simulink model "rlWalkingBipedRobot"  (R2023b)
settings: Solver=ode23t  StartTime=0.0  StopTime=inf  RelTol=1e-2  EnableMultiTasking=on
undefined symbols (not defined in the file): height_plane, init_angs_L, init_angs_R, init_height, joint_stiffness, lower_leg_length, max_torque, plane_x, plane_y, Tf, torso_offset_x, torso_offset_z, torso_x, torso_y, torso_z, Ts, upper_leg_length, wx0, wy0, X, Y, Z
libraries: sm_lib x27, nesl_utility x14, walkingRobotUtils x10, simulink x5, rllib x1
(part 2 of 2)

== system rlWalkingBipedRobot/Walking Robot/World and Ground ==
  Mechanism Configuration : sm_lib/Utilities/Mechanism Configuration  UniformGravity=Constant  GravityVector=[0 0 -9.80665]  GravityVectorUnits=m/s^2  LinearizationDelta=0.001  JointModeTransitionNonlinearIterations=2
  Plane Offset : sm_lib/Frames and Transforms/Rigid Transform  TranslationMethod=StandardAxis  TranslationStandardOffset=height_plane/2  TranslationStandardOffsetUnits=m  TranslationStandardAxis=-Z  TranslationCartesianOffset=[0 0 0]  TranslationCartesianOffsetUnits=m  TranslationROffset=0  TranslationROffsetUnits=m  TranslationZOffset=0  TranslationZOffsetUnits=m  TranslationThetaOffset=0  TranslationThetaOffsetUnits=deg  RotationMethod=None  RotationAngleUnits=deg  RotationStandardAxis=+Z  RotationAngle=0.0  RotationArbitraryAxis=[0 0 1]  FollAlignAxisA=+X  BaseAlignAxisA=+Y  FollAlignAxisB=+Y  BaseAlignAxisB=+Z  RotationSequenceAxes=FollowerAxes  RotationSequence=XYX  RotationSequenceAngles=[0 0 0]  RotationSequenceAnglesUnits=deg  RotationMatrix=[1 0 0; 0 1 0; 0 0 1]  Quaternion=[1 0 0 0]
  Solver Configuration : nesl_utility/Solver Configuration  PhysicalDomain=network_engine_domain  SubClassName=solver  LeftPortType=input  RightPortType=generic  Tones=[]  Harmonics=[]  SimulateNoise=off  Profile=off  UseLocalSampling=off  EnableSwitchedLinearOptims=on  FrequencyDomain=off  UseCCode=off  RelTol=0.001  AbsTol=1e-06  MinStep=1e-09  ToWorkspace=off  RevertToSquareIcSolve=off  NumHomotopyIterations=100  PhasorMode=off  PhasorModeNumHarmonics=1  ConsistencySolver=NEWTON_FTOL  IndexReductionMethod=DerivativeReplacement  DoDC=off  ResidualTolerance=1e-09  ConsistencyTolSource=GLOBAL  ConsistencyAbsTol=0.001  ConsistencyRelTol=0.001  ConsistencyTolFactor=0.001  UseLocalSolver=off  LocalSolverChoice=NE_TRAPEZOIDAL_ADVANCER  ResolveIndetEquations=on  FunctionEvalNumThread=1  LocalSolverSampleTime=Ts  DoFixedCost=off  MaxNonlinIter=3  MaxModeIter=2  ComputeImpulses=off  ImpulseIterations=2  LinearAlgebra=Sparse  LinearAlgebraNumThread=0  EquationFormulation=NE_TIME_EF  DelaysMemoryBudget=1024  AutomaticFiltering=on  FilteringTimeConstant=0.001  PartitionStorageMethod=AS_NEEDED  PartitionMemoryBudget=1024  PartitionMethod=FAST  MultibodyUseLocalSolver=off  MultibodyLocalSolverChoice=ODE1  MultibodyLocalSolverSampleTime=0.001
  World Frame1 : sm_lib/Frames and Transforms/World Frame
  World Plane : sm_lib/Body Elements/Brick Solid  GraphicAmbientColor=[0.15 0.15 0.15 1.0]  BasedOnType=Density  BrickDimensions="[plane_x plane_y  height_plane]"  BrickDimensionsUnits=m  CenterOfMass=[0 0 0]  CenterOfMassUnits=m  GraphicDiffuseColor=[1.0 1.0 0.8]  Density=density  DensityUnits=kg/(m^3)  DoExposeReferenceFrame=on  GraphicEmissiveColor=[0.0 0.0 0.0 1.0]  ExportEntireGeometry=on  SerializedFrames=<Frames/>  MarkerShape=Sphere  MarkerSize=10  GraphicType=FromGeometry  InertiaType=CalculateFromGeometry  Mass=1  MassUnits=kg  MomentsOfInertia=[1 1 1]  MomentsOfInertiaUnits=kg*m^2  GraphicOpacity=0.5  ProductsOfInertia=[0 0 0]  ProductsOfInertiaUnits=kg*m^2  GraphicShininess=75  GraphicSpecularColor=[0.5 0.5 0.5 1.0]  GraphicVisPropType=SimpleVisualProperties
  W : PMIOPort  Side=Left
  G : PMIOPort  Port=2  Side=Right
  connections:
  G/RConn1 -- World Plane/LConn1
  World Plane/RConn1 -- Plane Offset/RConn1
  Solver Configuration/RConn1 -- Plane Offset/LConn1 -- Mechanism Configuration/RConn1 -- W/RConn1 -- World Frame1/RConn1

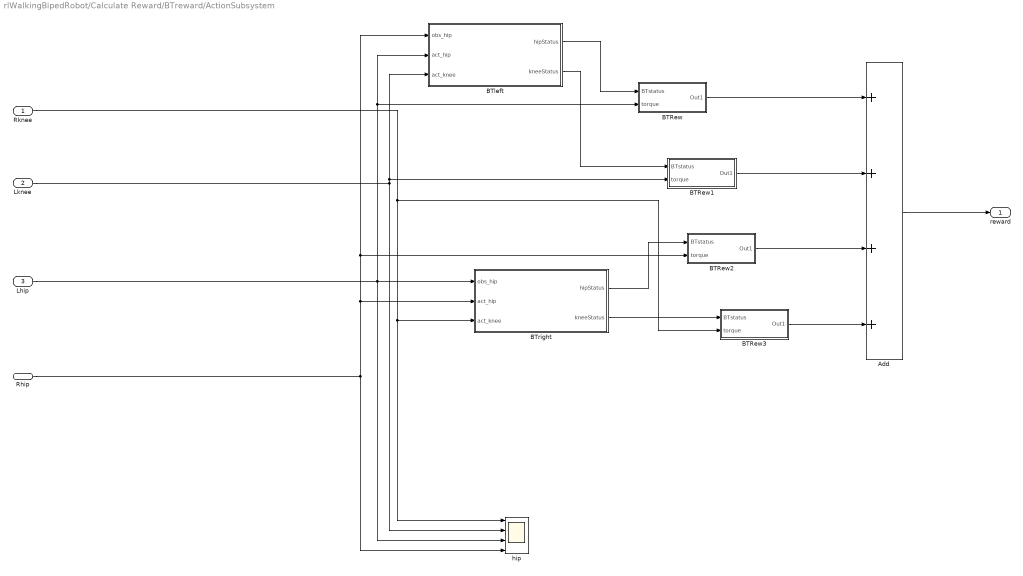
== system rlWalkingBipedRobot/Calculate Reward/BTreward/ActionSubsystem ==
  Rknee : Inport
  Lknee : Inport  Port=2
  Lhip : Inport  Port=3
  Rhip : Inport  Port=4
  Add : Sum  Inputs=++++
  BTRew : Subsystem
  BTRew1 : Subsystem
  BTRew2 : Subsystem
  BTRew3 : Subsystem
  BTleft : Subsystem
  BTright : Subsystem
  hip : Scope  NumInputPorts=4
  reward : Outport
  wires:
  Rknee/1 -> BTright/3(act_knee), hip/1, BTRew3/2(torque)
  Lknee/1 -> BTRew1/2(torque), BTleft/3(act_knee), hip/2
  Lhip/1 -> BTleft/2(act_hip), BTRew/2(torque), BTright/1(obs_hip), hip/3
  Rhip/1 -> BTRew2/2(torque), BTleft/1(obs_hip), BTright/2(act_hip), hip/4
  BTleft/1(hipStatus) -> BTRew/1(BTstatus)
  BTleft/2(kneeStatus) -> BTRew1/1(BTstatus)
  BTright/1(hipStatus) -> BTRew2/1(BTstatus)
  BTright/2(kneeStatus) -> BTRew3/1(BTstatus)
  BTRew/1(Out1) -> Add/1
  BTRew1/1(Out1) -> Add/2
  BTRew2/1(Out1) -> Add/3
  BTRew3/1(Out1) -> Add/4
  Add/1 -> reward/1

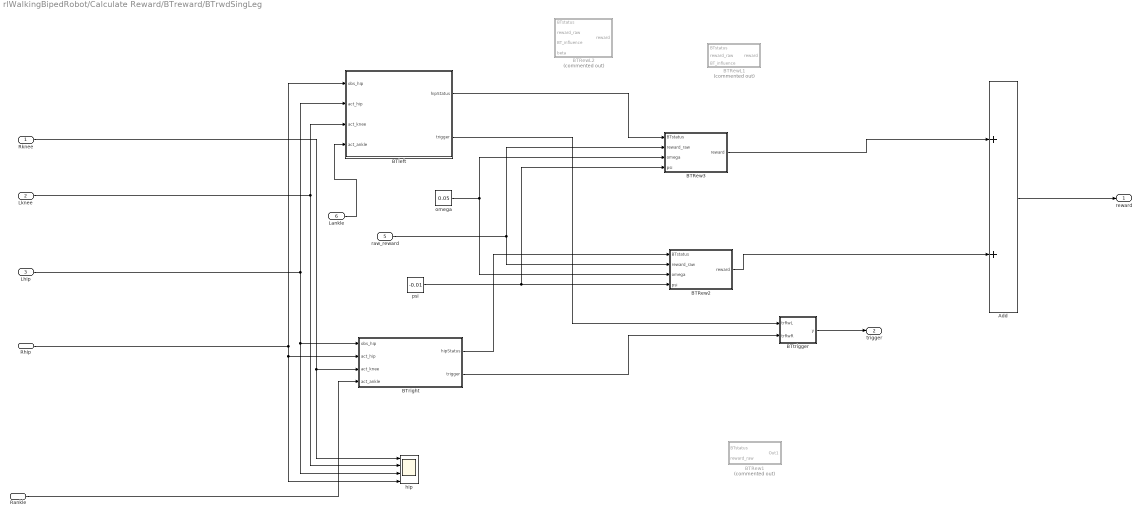
== system rlWalkingBipedRobot/Calculate Reward/BTreward/BTrwdSingLeg ==
  Rknee : Inport
  Lknee : Inport  Port=2
  Lhip : Inport  Port=3
  Rhip : Inport  Port=4
  raw_reward : Inport  Port=5
  Lankle : Inport  Port=6
  Rankle : Inport  Port=7
  Add : Sum
  BTRew1 : Subsystem  Commented=on
  BTRew2 : Subsystem
  BTRew3 : Subsystem
  BTRewL1 : Subsystem  Commented=on
  BTRewL2 : Subsystem  Commented=on
  BTleft : Subsystem
  BTright : Subsystem
  BTtrigger : MATLAB Function  TreatAsAtomicUnit=on
  hip : Scope  NumInputPorts=4
  omega : Constant  Value=0.05
  psi : Constant  Value=-0.01
  reward : Outport
  trigger : Outport  Port=2
  wires:
  Rknee/1 -> hip/1, BTright/3(act_knee)
  Lknee/1 -> BTleft/3(act_knee), hip/2
  Lhip/1 -> hip/3, BTright/1(obs_hip), BTleft/2(act_hip)
  Rhip/1 -> hip/4, BTright/2(act_hip), BTleft/1(obs_hip)
  BTRew3/1(reward) -> Add/1
  BTRew2/1(reward) -> Add/2
  Add/1 -> reward/1
  raw_reward/1 -> BTRew3/2(reward_raw), BTRew2/2(reward_raw)
  BTtrigger/1(y) -> trigger/1
  BTleft/1(hipStatus) -> BTRew3/1(BTstatus)
  BTright/1(hipStatus) -> BTRew2/1(BTstatus)
  BTleft/2(trigger) -> BTtrigger/1(trRwL)
  BTright/2(trigger) -> BTtrigger/2(trRwR)
  Rankle/1 -> BTright/4(act_ankle)
  Lankle/1 -> BTleft/4(act_ankle)
  omega/1 -> BTRew3/3(omega), BTRew2/3(omega)
  psi/1 -> BTRew3/4(psi), BTRew2/4(psi)

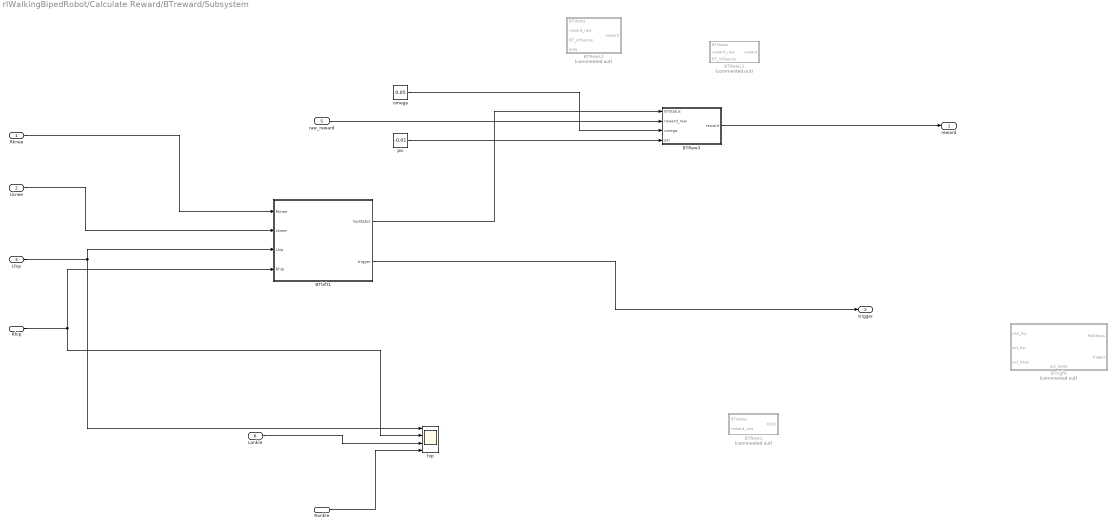
== system rlWalkingBipedRobot/Calculate Reward/BTreward/Subsystem ==
  Rknee : Inport
  Lknee : Inport  Port=2
  Lhip : Inport  Port=3
  Rhip : Inport  Port=4
  raw_reward : Inport  Port=5
  Lankle : Inport  Port=6
  Rankle : Inport  Port=7
  BTRew1 : Subsystem  Commented=on
  BTRew3 : Subsystem
  BTRewL1 : Subsystem  Commented=on
  BTRewL2 : Subsystem  Commented=on
  BTleft1 : Subsystem
  BTright : Subsystem  Commented=on
      settings: PortSchema="{\"entries\":[{\"content\":{\"sides\":[{\"content\":{\"connectorIds\":[\"In1\",\"In2\",\"In3\"]},\"type\":\"ConnectorPlacement.EquallySpacedRectSide\",\"uuid\":\"d1a7c831-0d82-4d6a-8038-37bdddb40f4b\"},{\"content\":{\"connectorIds\":[\"Out1\",\"Out2\"],\"side\":\"RIGHT\"},\"type\":\"ConnectorPlacement.EquallySpacedRectSide\",\"uuid\":\"e646f7d3-ea41-40b5-b80d-dc533f9acebb\"},{\"content\":{\"side\":\"TOP\"},\"type\":\"ConnectorPlacement.EquallySpacedRectSide\",\"uuid\":\"96bfc05b-3d35-40ea-a71c-eb204fc643e2\"},{\"content\":{\"connectorIds\":[\"In4\"],\"side\":\"BOTTOM\"},\"type\":\"ConnectorPlacement.EquallySpacedRectSide\",\"uuid\":\"1094da1b-3afd-404e-9933-6191ea7e4b5f\"}]},\"type\":\"ConnectorPlacement.EquallySpacedConnector\",\"uuid\":\"abf6e411-f407-44d6-9c89-b64076b2e2db\"}],\"packageUris\":[\"http://schema.mathworks.com/mf0/Connector/R2020b\"],\"version\":\"1.0\"}"
  hip : Scope  NumInputPorts=4
  omega : Constant  Value=0.05
  psi : Constant  Value=-0.01
  reward : Outport
  trigger : Outport  Port=2
  wires:
  Rknee/1 -> BTleft1/1(Rknee)
  Lknee/1 -> BTleft1/2(Lknee)
  Lhip/1 -> hip/1, BTleft1/3(Lhip)
  Rhip/1 -> hip/2, BTleft1/4(Rhip)
  BTRew3/1(reward) -> reward/1
  raw_reward/1 -> BTRew3/2(reward_raw)
  BTleft1/2(trigger) -> trigger/1
  Lankle/1 -> hip/3
  omega/1 -> BTRew3/3(omega)
  psi/1 -> BTRew3/4(psi)
  BTleft1/1(hipStatus) -> BTRew3/1(BTstatus)
  Rankle/1 -> hip/4

== system rlWalkingBipedRobot/Walking Robot/Sensors/Calculate Actuator Power ==
  meas : Inport
  Add : Sum  Inputs=3
  Bus Selector : BusSelector  OutputSignals=ankle_speed,ankle_torque,knee_speed,knee_torque,hip_speed,hip_torque
  Product : Product
  Product1 : Product
  Product2 : Product
  P : Outport  VectorParamsAs1DForOutWhenUnconnected=off
  wires:
  meas/1 -> Bus Selector/1
  Product2/1 -> Add/3
  Product1/1 -> Add/2
  Product/1 -> Add/1
  Add/1 -> P/1
  Bus Selector/1 -> Product/1  "<ankle_speed>"
  Bus Selector/2 -> Product/2  "<ankle_torque>"
  Bus Selector/3 -> Product1/1  "<knee_speed>"
  Bus Selector/4 -> Product1/2  "<knee_torque>"
  Bus Selector/5 -> Product2/1  "<hip_speed>"
  Bus Selector/6 -> Product2/2  "<hip_torque>"

== system rlWalkingBipedRobot/Walking Robot/Sensors/Calculate Actuator Power1 ==
  meas : Inport
  Add : Sum  Inputs=3
  Bus Selector : BusSelector  OutputSignals=ankle_speed,ankle_torque,knee_speed,knee_torque,hip_speed,hip_torque
  Product : Product
  Product1 : Product
  Product2 : Product
  P : Outport  VectorParamsAs1DForOutWhenUnconnected=off
  wires:
  Bus Selector/6 -> Product2/2  "<hip_torque>"
  Bus Selector/5 -> Product2/1  "<hip_speed>"
  Bus Selector/4 -> Product1/2  "<knee_torque>"
  Bus Selector/3 -> Product1/1  "<knee_speed>"
  Bus Selector/2 -> Product/2  "<ankle_torque>"
  Bus Selector/1 -> Product/1  "<ankle_speed>"
  Add/1 -> P/1
  Product/1 -> Add/1
  Product1/1 -> Add/2
  Product2/1 -> Add/3
  meas/1 -> Bus Selector/1

== system rlWalkingBipedRobot/Calculate Reward/BTreward/ActionSubsystem/BTRew ==
  BTstatus : Inport
  torque : Inport  Port=2
  Abs : Abs  SaturateOnIntegerOverflow=off
  Gain : Gain  Gain=0.1
  Product : Product
  Out1 : Outport
  wires:
  Gain/1 -> Out1/1
  torque/1 -> Abs/1
  Abs/1 -> Product/2
  Product/1 -> Gain/1
  BTstatus/1 -> Product/1

== system rlWalkingBipedRobot/Calculate Reward/BTreward/ActionSubsystem/BTRew1 ==
  BTstatus : Inport
  torque : Inport  Port=2
  Abs : Abs  SaturateOnIntegerOverflow=off
  Gain : Gain  Gain=0.1
  Product : Product
  Out1 : Outport
  wires:
  Gain/1 -> Out1/1
  torque/1 -> Abs/1
  Abs/1 -> Product/2
  Product/1 -> Gain/1
  BTstatus/1 -> Product/1

== system rlWalkingBipedRobot/Calculate Reward/BTreward/ActionSubsystem/BTRew2 ==
  BTstatus : Inport
  torque : Inport  Port=2
  Abs : Abs  SaturateOnIntegerOverflow=off
  Gain : Gain  Gain=0.1
  Product : Product
  Out1 : Outport
  wires:
  Gain/1 -> Out1/1
  torque/1 -> Abs/1
  Abs/1 -> Product/2
  Product/1 -> Gain/1
  BTstatus/1 -> Product/1

== system rlWalkingBipedRobot/Calculate Reward/BTreward/ActionSubsystem/BTRew3 ==
  BTstatus : Inport
  torque : Inport  Port=2
  Abs : Abs  SaturateOnIntegerOverflow=off
  Gain : Gain  Gain=0.1
  Product : Product
  Out1 : Outport
  wires:
  Gain/1 -> Out1/1
  torque/1 -> Abs/1
  Abs/1 -> Product/2
  Product/1 -> Gain/1
  BTstatus/1 -> Product/1

== system rlWalkingBipedRobot/Calculate Reward/BTreward/ActionSubsystem/BTleft ==
  obs_hip : Inport
  act_hip : Inport  Port=2
  act_knee : Inport  Port=3
  BT : MATLAB Function  TreatAsAtomicUnit=on
  hipStatus : Outport
  kneeStatus : Outport  Port=2
  wires:
  obs_hip/1 -> BT/1(u)
  BT/1(y) -> hipStatus/1
  act_hip/1 -> BT/2(t)
  act_knee/1 -> BT/3(s)
  BT/2(z) -> kneeStatus/1

== system rlWalkingBipedRobot/Calculate Reward/BTreward/ActionSubsystem/BTright ==
  obs_hip : Inport
  act_hip : Inport  Port=2
  act_knee : Inport  Port=3
  BT : MATLAB Function  TreatAsAtomicUnit=on
  hipStatus : Outport
  kneeStatus : Outport  Port=2
  wires:
  obs_hip/1 -> BT/1(u)
  BT/1(y) -> hipStatus/1
  act_hip/1 -> BT/2(t)
  act_knee/1 -> BT/3(s)
  BT/2(z) -> kneeStatus/1

== system rlWalkingBipedRobot/Calculate Reward/BTreward/BTrwdSingLeg/BTRew1 ==
  BTstatus : Inport
  reward_raw : Inport  Port=2
  Product1 : Product
  rew2BT : MATLAB Function  TreatAsAtomicUnit=on
  Out1 : Outport
  wires:
  Product1/1 -> Out1/1
  BTstatus/1 -> Product1/1
  reward_raw/1 -> rew2BT/1(x)
  rew2BT/1(y) -> Product1/2

== system rlWalkingBipedRobot/Calculate Reward/BTreward/BTrwdSingLeg/BTRew2 ==
  BTstatus : Inport
  reward_raw : Inport  Port=2
  omega : Inport  Port=3
  psi : Inport  Port=4
  rew2BT : MATLAB Function  TreatAsAtomicUnit=on
  reward : Outport
  wires:
  rew2BT/1(y) -> reward/1
  BTstatus/1 -> rew2BT/3(BTstatus)
  reward_raw/1 -> rew2BT/4(x)
  omega/1 -> rew2BT/1(omega)
  psi/1 -> rew2BT/2(psi)

== system rlWalkingBipedRobot/Calculate Reward/BTreward/BTrwdSingLeg/BTRew3 ==
  BTstatus : Inport
  reward_raw : Inport  Port=2
  omega : Inport  Port=3
  psi : Inport  Port=4
  rew2BT : MATLAB Function  TreatAsAtomicUnit=on
  reward : Outport
  wires:
  rew2BT/1(y) -> reward/1
  BTstatus/1 -> rew2BT/3(BTstatus)
  reward_raw/1 -> rew2BT/4(x)
  omega/1 -> rew2BT/1(omega)
  psi/1 -> rew2BT/2(psi)

== system rlWalkingBipedRobot/Calculate Reward/BTreward/BTrwdSingLeg/BTRewL1 ==
  BTstatus : Inport
  reward_raw : Inport  Port=2
  BT_influence : Inport  Port=3
  Product1 : Product
  rew2BT : MATLAB Function  TreatAsAtomicUnit=on
  reward : Outport
  wires:
  Product1/1 -> reward/1
  BTstatus/1 -> Product1/1
  reward_raw/1 -> rew2BT/1(x)
  rew2BT/1(y) -> Product1/2
  BT_influence/1 -> rew2BT/2(alfa)

== system rlWalkingBipedRobot/Calculate Reward/BTreward/BTrwdSingLeg/BTRewL2 ==
  BTstatus : Inport
  reward_raw : Inport  Port=2
  BT_influence : Inport  Port=3
  beta : Inport  Port=4
  Product1 : Product
  rew2BT : MATLAB Function  TreatAsAtomicUnit=on
  reward : Outport
  wires:
  Product1/1 -> reward/1
  BTstatus/1 -> Product1/1
  reward_raw/1 -> rew2BT/1(x)
  rew2BT/1(y) -> Product1/2
  BT_influence/1 -> rew2BT/2(alfa)
  beta/1 -> rew2BT/3(beta)

== system rlWalkingBipedRobot/Calculate Reward/BTreward/BTrwdSingLeg/BTleft ==
  obs_hip : Inport
  act_hip : Inport  Port=2
  act_knee : Inport  Port=3
  act_ankle : Inport  Port=4
  BT : MATLAB Function  TreatAsAtomicUnit=on
  hipStatus : Outport
  trigger : Outport  Port=2
  wires:
  obs_hip/1 -> BT/1(u)
  BT/1(y) -> hipStatus/1
  act_hip/1 -> BT/2(h)
  act_knee/1 -> BT/3(k)
  BT/2(trigger) -> trigger/1
  act_ankle/1 -> BT/4(a)

== system rlWalkingBipedRobot/Calculate Reward/BTreward/BTrwdSingLeg/BTright ==
  obs_hip : Inport
  act_hip : Inport  Port=2
  act_knee : Inport  Port=3
  act_ankle : Inport  Port=4
  BT : MATLAB Function  TreatAsAtomicUnit=on
  hipStatus : Outport
  trigger : Outport  Port=2
  wires:
  obs_hip/1 -> BT/1(u)
  BT/1(y) -> hipStatus/1
  act_hip/1 -> BT/2(h)
  act_knee/1 -> BT/3(k)
  BT/2(trigger) -> trigger/1
  act_ankle/1 -> BT/4(a)

== system rlWalkingBipedRobot/Calculate Reward/BTreward/Subsystem/BTRew1 ==
  BTstatus : Inport
  reward_raw : Inport  Port=2
  Product1 : Product
  rew2BT : MATLAB Function  TreatAsAtomicUnit=on
  Out1 : Outport
  wires:
  Product1/1 -> Out1/1
  BTstatus/1 -> Product1/1
  reward_raw/1 -> rew2BT/1(x)
  rew2BT/1(y) -> Product1/2

== system rlWalkingBipedRobot/Calculate Reward/BTreward/Subsystem/BTRew3 ==
  BTstatus : Inport
  reward_raw : Inport  Port=2
  omega : Inport  Port=3
  psi : Inport  Port=4
  rew2BT : MATLAB Function  TreatAsAtomicUnit=on
  reward : Outport
  wires:
  rew2BT/1(y) -> reward/1
  BTstatus/1 -> rew2BT/3(BTstatus)
  reward_raw/1 -> rew2BT/4(x)
  omega/1 -> rew2BT/1(omega)
  psi/1 -> rew2BT/2(psi)

== system rlWalkingBipedRobot/Calculate Reward/BTreward/Subsystem/BTRewL1 ==
  BTstatus : Inport
  reward_raw : Inport  Port=2
  BT_influence : Inport  Port=3
  Product1 : Product
  rew2BT : MATLAB Function  TreatAsAtomicUnit=on
  reward : Outport
  wires:
  Product1/1 -> reward/1
  BTstatus/1 -> Product1/1
  reward_raw/1 -> rew2BT/1(x)
  rew2BT/1(y) -> Product1/2
  BT_influence/1 -> rew2BT/2(alfa)

== system rlWalkingBipedRobot/Calculate Reward/BTreward/Subsystem/BTRewL2 ==
  BTstatus : Inport
  reward_raw : Inport  Port=2
  BT_influence : Inport  Port=3
  beta : Inport  Port=4
  Product1 : Product
  rew2BT : MATLAB Function  TreatAsAtomicUnit=on
  reward : Outport
  wires:
  Product1/1 -> reward/1
  BTstatus/1 -> Product1/1
  reward_raw/1 -> rew2BT/1(x)
  rew2BT/1(y) -> Product1/2
  BT_influence/1 -> rew2BT/2(alfa)
  beta/1 -> rew2BT/3(beta)

== system rlWalkingBipedRobot/Calculate Reward/BTreward/Subsystem/BTleft1 ==
  Rknee : Inport
  Lknee : Inport  Port=2
  Lhip : Inport  Port=3
  Rhip : Inport  Port=4
  BTandRw : MATLAB Function  TreatAsAtomicUnit=on
  hipStatus : Outport
  trigger : Outport  Port=2
  wires:
  Rknee/1 -> BTandRw/1(RK)
  BTandRw/1(BTstatus) -> hipStatus/1
  Rhip/1 -> BTandRw/2(RH)
  Lknee/1 -> BTandRw/3(LK)
  BTandRw/2(trigger) -> trigger/1
  Lhip/1 -> BTandRw/4(LH)

== system rlWalkingBipedRobot/Calculate Reward/BTreward/Subsystem/BTright ==
  obs_hip : Inport
  act_hip : Inport  Port=2
  act_knee : Inport  Port=3
  act_ankle : Inport  Port=4
  BT : MATLAB Function  TreatAsAtomicUnit=on
  hipStatus : Outport
  trigger : Outport  Port=2
  wires:
  obs_hip/1 -> BT/1(u)
  BT/1(y) -> hipStatus/1
  act_hip/1 -> BT/2(h)
  act_knee/1 -> BT/3(k)
  BT/2(trigger) -> trigger/1
  act_ankle/1 -> BT/4(a)

== matlab function rlWalkingBipedRobot/Calculate Reward/BTreward/BTrwdSingLeg/BTRew1/rew2BT ==
  data: x input; y output
function y = fcn(x)
y = -1.5 + 1/(1 + exp(-x)) + (1 - tanh(x))*x/2;

== matlab function rlWalkingBipedRobot/Calculate Reward/BTreward/BTrwdSingLeg/BTRew2/rew2BT ==
  data: omega input; psi input; BTstatus input; x input; y output
function y = fcn(omega, psi, BTstatus, x)
if BTstatus > 0.1 %adding .1 to be sure to not take l=value slightly higher than 0
    if omega*x < psi
        y = omega*x;
    else
        y= psi;
    end
else
    y = 0.0;
end


%function y = fcn(omega_in, psi, signal, x)

%alfa = signal*alfa_in;


%y = beta + (alfa*x - beta)/(1 + exp(x+2))
% y = -1.5 + 1/(1 + exp(-x)) + (1 - tanh(x))*x/2;

== matlab function rlWalkingBipedRobot/Walking Robot/Sensors/Rotation Matrix to Yaw Pitch Roll ==
  data: q input; eul output
function eul = calcAttitude(q)

% Normalize the quaternions
q = bsxfun(@times, q, 1./sqrt(sum(q.^2,1)));
qw = q(1);
qx = q(2);
qy = q(3);
qz = q(4);

% Pre-allocate output
eul = zeros(3, 1, 'like', q);

aSinInput = -2*(qx.*qz-qw.*qy);
aSinInput(aSinInput > 1) = 1;
aSinInput(aSinInput < -1) = -1;

eul = [ atan2( 2*(qx.*qy+qw.*qz), qw.^2 + qx.^2 - qy.^2 - qz.^2 ); ...
    asin( aSinInput ); ...
    atan2( 2*(qy.*qz+qw.*qx), qw.^2 - qx.^2 - qy.^2 + qz.^2 )];

== matlab function rlWalkingBipedRobot/Calculate Reward/BTreward/BTrwdSingLeg/BTRew3/rew2BT ==
  data: omega input; psi input; BTstatus input; x input; y output
function y = fcn(omega, psi, BTstatus, x)
if BTstatus > 0.1 %adding .1 to be sure to not take l=value slightly higher than 0
    if omega*x < psi
        y = omega*x;
    else
        y= psi;
    end
else
    y = 0.0;
end


%function y = fcn(omega_in, psi, signal, x)

%alfa = signal*alfa_in;


%y = beta + (alfa*x - beta)/(1 + exp(x+2))
% y = -1.5 + 1/(1 + exp(-x)) + (1 - tanh(x))*x/2;

== matlab function rlWalkingBipedRobot/Calculate Reward/BTreward/BTrwdSingLeg/BTRewL1/rew2BT ==
  data: x input; y output; alfa input
function y= fcn(x,alfa)
% trigger = 0;
% y = 0;
% thresholdBT = 0.511972; % x+alfa*(1/(1+e^(-x)) + (1-tanh(x))*x/2-1) + beta =0
% tolThreshBT = 0.2*thresholdBT;
% if ((x<0-tolThreshBT) || (x>thresholdBT+tolThreshBT))
%     beta = -0.5;
%     y = beta + alfa*(1/(1 + exp(-x)) + (1 - tanh(x))*x/2 - 1);
%     trigger = 10;
%end
beta = -0.5;
y = beta + alfa*(1/(1 + exp(-x)) + (1 - tanh(x))*x/2 - 1);

== matlab function rlWalkingBipedRobot/Calculate Reward/BTreward/BTrwdSingLeg/BTRewL2/rew2BT ==
  data: x input; y output; alfa input; beta input
function y= fcn(x,alfa, beta)
% trigger = 0;
% y = 0;
% thresholdBT = 0.511972; % x+alfa*(1/(1+e^(-x)) + (1-tanh(x))*x/2-1) + beta =0
% tolThreshBT = 0.2*thresholdBT;
% if ((x<0-tolThreshBT) || (x>thresholdBT+tolThreshBT))
%     beta = -0.5;
%     y = beta + alfa*(1/(1 + exp(-x)) + (1 - tanh(x))*x/2 - 1);
%     trigger = 10;
%end
y = beta + alfa*(1/(1 + exp(-x)) + (1 - tanh(x))*x/2 - 1);

== matlab function rlWalkingBipedRobot/Calculate Reward/BTreward/BTrwdSingLeg/BTleft/BT ==
  data: u input; y output; h input; k input; trigger output; a input
function [y, trigger]= fcn(u,h,k,a)
y = 0;
trigger = 0;
if (u<0)
    if (h<0 || k<0) % hips moving on the same sense
        y = 1;
        trigger = 10;
    end
elseif (u>0)
    if (h>0 || k>0) % legs moving on the same sense
        y = 1;
        trigger = 10;
    end
end

== matlab function rlWalkingBipedRobot/Calculate Reward/BTreward/BTrwdSingLeg/BTright/BT ==
  data: u input; y output; h input; k input; trigger output; a input
function [y, trigger]= fcn(u,h,k,a)
y = 0;
trigger = 0;
if (u<0)
    if (h<0) % hips moving on the same sense
        y = 1;
        trigger = 10;
    end
elseif (u>0)
    if (h>0) % legs moving on the same sense
        y = 1;
        trigger = 10;
    end
end

== matlab function rlWalkingBipedRobot/Calculate Reward/BTreward/BTrwdSingLeg/BTtrigger ==
  data: trRwL input; y output; trRwR input
function y = fcn(trRwL,trRwR)
y = 0;
if (trRwL>5)
    y=10;
end
if (trRwR>5)
    y=10;
end

== matlab function rlWalkingBipedRobot/Calculate Reward/BTreward/Subsystem/BTleft1/BTandRw ==
  data: RK input; BTstatus output; RH input; LK input; LH input; trigger output
function [BTstatus, trigger]= fcn(RK, RH, LK, LH)
trigger = 0;
if ((RH >= 0 && LH <= 0 ) || ...
        (RH <= 0 && LH >= 0)) % all good
    BTstatus = 0;
    trigger = 0;
else % all bad
    BTstatus = 1;
    trigger = 10;
end

== matlab function rlWalkingBipedRobot/Calculate Reward/BTreward/Subsystem/BTright/BT ==
  data: u input; y output; h input; k input; trigger output; a input
function [y, trigger]= fcn(u,h,k,a)
y = 0;
trigger = 0;
if (u<0)
    if (h<0) % hips moving on the same sense
        y = 1;
        trigger = 10;
    end
elseif (u>0)
    if (h>0) % legs moving on the same sense
        y = 1;
        trigger = 10;
    end
end

== matlab function rlWalkingBipedRobot/Calculate Reward/BTreward/ActionSubsystem/BTleft/BT ==
  data: u input; y output; t input; s input; z output
function [y,z]= fcn(u,t,s)
y = 0;
z = 0;
if (u<0)
    if (t<0) % hips moving on the same sense
        y = -1;
    end
    if (s<0) % knee moving on the wrong sense
        z = -1;
    end
elseif (u>0)
    if (t>0) % legs moving on the same sense
        y = -1;
    end
    if (s>0) % knee moving on the wrong sense
        z = -1;
    end
end

== matlab function rlWalkingBipedRobot/Calculate Reward/BTreward/ActionSubsystem/BTright/BT ==
  data: u input; y output; t input; s input; z output
function [y,z]= fcn(u,t,s)
y = 0;
z = 0;
if (u<0)
    if (t<0) % hips moving on the same sense
        y = -1;
    end
    %if (s<0) % knee moving on the wrong sense
    %    z = -1;
    %end
elseif (u>0)
    if (t>0) % legs moving on the same sense
        y = -1;
    end
    %if (s>0) % knee moving on the wrong sense
    %    z = -1;
    %end
end

== matlab function rlWalkingBipedRobot/Calculate Reward/BTreward/Subsystem/BTRewL1/rew2BT ==
  data: x input; y output; alfa input
function y= fcn(x,alfa)
% trigger = 0;
% y = 0;
% thresholdBT = 0.511972; % x+alfa*(1/(1+e^(-x)) + (1-tanh(x))*x/2-1) + beta =0
% tolThreshBT = 0.2*thresholdBT;
% if ((x<0-tolThreshBT) || (x>thresholdBT+tolThreshBT))
%     beta = -0.5;
%     y = beta + alfa*(1/(1 + exp(-x)) + (1 - tanh(x))*x/2 - 1);
%     trigger = 10;
%end
beta = -0.5;
y = beta + alfa*(1/(1 + exp(-x)) + (1 - tanh(x))*x/2 - 1);

== matlab function rlWalkingBipedRobot/Calculate Reward/BTreward/Subsystem/BTRew3/rew2BT ==
  data: omega input; psi input; BTstatus input; x input; y output
function y = fcn(omega, psi, BTstatus, x)
if BTstatus > 0.1 %adding .1 to be sure to not take l=value slightly higher than 0
    if omega*x < psi
        y = omega*x;
    else
        y= psi;
    end
else
    y = 0.0;
end


%function y = fcn(omega_in, psi, signal, x)

%alfa = signal*alfa_in;


%y = beta + (alfa*x - beta)/(1 + exp(x+2))
% y = -1.5 + 1/(1 + exp(-x)) + (1 - tanh(x))*x/2;

== matlab function rlWalkingBipedRobot/Calculate Reward/BTreward/Subsystem/BTRew1/rew2BT ==
  data: x input; y output
function y = fcn(x)
y = -1.5 + 1/(1 + exp(-x)) + (1 - tanh(x))*x/2;

== matlab function rlWalkingBipedRobot/Calculate Reward/MATLAB Function1 ==
  data: defaultReward input; y output; trigger input; BTreward input
function y = fcn(defaultReward, trigger, BTreward)
%#codegen

y = defaultReward;

if (trigger > 5)
    y = y+BTreward;
end

== matlab function rlWalkingBipedRobot/Calculate Reward/BTreward/Subsystem/BTRewL2/rew2BT ==
  data: x input; y output; alfa input; beta input
function y= fcn(x,alfa, beta)
% trigger = 0;
% y = 0;
% thresholdBT = 0.511972; % x+alfa*(1/(1+e^(-x)) + (1-tanh(x))*x/2-1) + beta =0
% tolThreshBT = 0.2*thresholdBT;
% if ((x<0-tolThreshBT) || (x>thresholdBT+tolThreshBT))
%     beta = -0.5;
%     y = beta + alfa*(1/(1 + exp(-x)) + (1 - tanh(x))*x/2 - 1);
%     trigger = 10;
%end
y = beta + alfa*(1/(1 + exp(-x)) + (1 - tanh(x))*x/2 - 1);
